simulink model "AXI_QPSK_Tx"  (R2020a)
settings: Solver=FixedStepAuto  StartTime=0.0  StopTime=1000/Rb  RelTol=1e-3
PreLoadFcn:
  | Rb = 1000;   % 1kbit / s
  | Rsym = Rb/2;   % 2 bits per symbol
  | Rsymbol = Rb/2;
  | OSR = 32;
  | f_error = 120;
  | 
  | design_filters_tx
undefined symbols (not defined in the file or in its folder): AXI4, CIC_fine_Tx, fCIC, fHB, Lite, R_CIC, R_CICcomp, R_HB, R_RRC
libraries: xbsIndex_r4 x281, hdlsllib x2
(part 1 of 3)
CloseFcn:
  | clear
settings Model: Creator=nas07122  LastModifiedBy=david
settings DataIOCC: ReturnWorkspaceOutputs=off
settings DebuggingCC: ArithmeticOperatorsInVariantConditions=warning
settings SFSimCC: SimUseLocalCustomCode=off  CustomCodeUndefinedFunction=UseInterfaceOnly
settings RTWCC: RTWUseLocalCustomCode=off
settings CodeAppCC: StateflowObjectComments=on

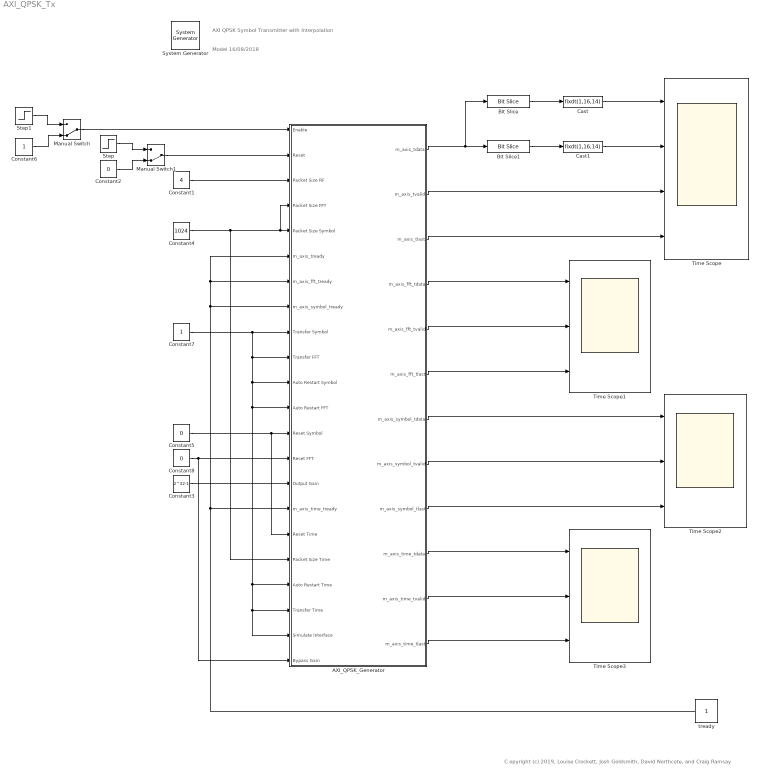
== system AXI_QPSK_Tx ==
  note: Model 16/08/2018
  note: AXI QPSK Symbol Transmitter with Interpolation
  note: C opyright (c) 2019, Louise Crockett, Josh Goldsmith, David Northcote, and Craig Ramsay
  " System Generator" : xbsIndex_r4/ System Generator  Tag=genX  xilinxfamily=zynquplusRFSOC  part=xczu28dr  speed=-2-e  package=ffvg1517  synthesis_tool=Vivado  clock_wrapper=Clock Enables  directory=../iprepo/zcu111/tx  proj_type=Vivado  Synth_file=Vivado Synthesis Defaults  Impl_file=Vivado Implementation Defaults  testbench=off  simulink_period=1/(0.5*Rb*R_RRC*R_HB*R_CICcomp*R_CIC)  sysclk_period=(1/fCIC)*1e9  dcm_input_clock_period=10  incr_netlist=off  trim_vbits=Everywhere in SubSystem  dbl_ovrd=According to Block Masks  core_generation=According to Block Masks  run_coregen=off  deprecated_control=off  eval_field=0  block_type=sysgen
  AXI_QPSK_Generator : Subsystem
  Bit Slice : hdlsllib/Logic and Bit Operations/Bit Slice  lidx=15  ridx=0
      settings: SourceProductBaseCode=SL
  Bit Slice1 : hdlsllib/Logic and Bit Operations/Bit Slice  lidx=31  ridx=16
      settings: SourceProductBaseCode=SL
  Cast : DataTypeConversion  OutDataTypeStr=fixdt(1,16,14)  ConvertRealWorld=Stored Integer (SI)
  Cast1 : DataTypeConversion  OutDataTypeStr=fixdt(1,16,14)  ConvertRealWorld=Stored Integer (SI)
  Constant1 : Constant  Value=4  SampleTime=2/Rb
  Constant2 : Constant  Value=0  SampleTime=2/Rb
  Constant3 : Constant  Value=2^32-1  SampleTime=1/fHB
  Constant4 : Constant  Value=1024  SampleTime=1/fCIC
  Constant5 : Constant  Value=0  SampleTime=1/fCIC
  Constant6 : Constant  SampleTime=2/Rb
  Constant7 : Constant  SampleTime=1/fCIC
  Constant8 : Constant  Value=0  SampleTime=1/fHB
  Manual Switch : ManualSwitch  CurrentSetting=0
  Manual Switch1 : ManualSwitch  CurrentSetting=0
  Step : Step  Time=5/Rb  Before=1  After=0  SampleTime=2/Rb
  Step1 : Step  Time=8/Rb  SampleTime=2/Rb
  Time Scope : Scope  NumInputPorts=4
  Time Scope1 : Scope  NumInputPorts=3
  Time Scope2 : Scope  NumInputPorts=3
  Time Scope3 : Scope  NumInputPorts=3
  tready : Constant  VectorParams1D=off  OutDataTypeStr=boolean  SampleTime=-1
  wires:
  Step1/1 -> Manual Switch/1
  Constant6/1 -> Manual Switch/2
  Bit Slice/1 -> Cast/1
  Bit Slice1/1 -> Cast1/1
  AXI_QPSK_Generator/1(m_axis_tdata) -> Bit Slice/1, Bit Slice1/1
  Manual Switch/1 -> AXI_QPSK_Generator/1(Enable)
  Constant1/1 -> AXI_QPSK_Generator/3(Packet Size RF)
  tready/1 -> AXI_QPSK_Generator/6(m_axis_tready), AXI_QPSK_Generator/7(m_axis_fft_tready), AXI_QPSK_Generator/8(m_axis_symbol_tready), AXI_QPSK_Generator/16(m_axis_time_tready)
  AXI_QPSK_Generator/2(m_axis_tvalid) -> Time Scope/3
  AXI_QPSK_Generator/3(m_axis_tlast) -> Time Scope/4
  Cast1/1 -> Time Scope/2
  Cast/1 -> Time Scope/1
  Manual Switch1/1 -> AXI_QPSK_Generator/2(Reset)
  Step/1 -> Manual Switch1/1
  Constant2/1 -> Manual Switch1/2
  Constant4/1 -> AXI_QPSK_Generator/4(Packet Size FFT), AXI_QPSK_Generator/5(Packet Size Symbol), AXI_QPSK_Generator/18(Packet Size Time)
  AXI_QPSK_Generator/7(m_axis_symbol_tdata) -> Time Scope2/1
  AXI_QPSK_Generator/8(m_axis_symbol_tvalid) -> Time Scope2/2
  AXI_QPSK_Generator/9(m_axis_symbol_tlast) -> Time Scope2/3
  AXI_QPSK_Generator/6(m_axis_fft_tlast) -> Time Scope1/3
  AXI_QPSK_Generator/5(m_axis_fft_tvalid) -> Time Scope1/2
  AXI_QPSK_Generator/4(m_axis_fft_tdata) -> Time Scope1/1
  Constant5/1 -> AXI_QPSK_Generator/17(Reset Time), AXI_QPSK_Generator/13(Reset Symbol)
  Constant7/1 -> AXI_QPSK_Generator/21(Simulate Interface), AXI_QPSK_Generator/20(Transfer Time), AXI_QPSK_Generator/19(Auto Restart Time), AXI_QPSK_Generator/12(Auto Restart FFT), AXI_QPSK_Generator/11(Auto Restart Symbol), AXI_QPSK_Generator/10(Transfer FFT), AXI_QPSK_Generator/9(Transfer Symbol)
  Constant8/1 -> AXI_QPSK_Generator/22(Bypass Gain), AXI_QPSK_Generator/14(Reset FFT)
  AXI_QPSK_Generator/10(m_axis_time_tdata) -> Time Scope3/1
  AXI_QPSK_Generator/11(m_axis_time_tvalid) -> Time Scope3/2
  AXI_QPSK_Generator/12(m_axis_time_tlast) -> Time Scope3/3
  Constant3/1 -> AXI_QPSK_Generator/15(Output Gain)

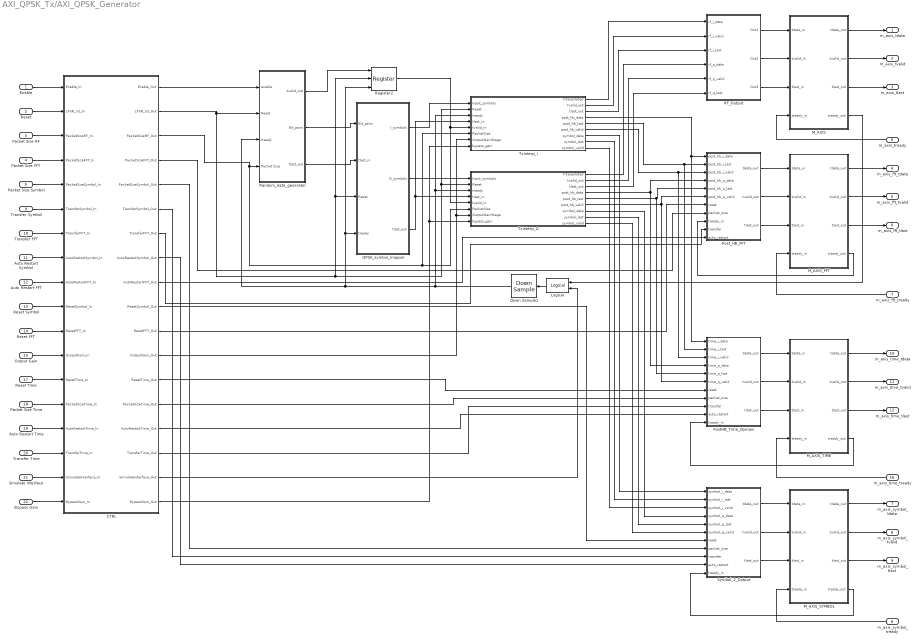
== system AXI_QPSK_Tx/AXI_QPSK_Generator ==
  Enable : Inport
  Reset : Inport  Port=2
  Packet Size RF : Inport  Port=3
  Packet Size FFT : Inport  Port=4
  Packet Size Symbol : Inport  Port=5
  m_axis_tready : Inport  Port=6
  m_axis_fft_tready : Inport  Port=7
  m_axis_symbol_tready : Inport  Port=8
  Transfer Symbol : Inport  Port=9
  Transfer FFT : Inport  Port=10
  Auto Restart Symbol : Inport  Port=11
  Auto Restart FFT : Inport  Port=12
  Reset Symbol : Inport  Port=13
  Reset FFT : Inport  Port=14
  Output Gain : Inport  Port=15
  m_axis_time_tready : Inport  Port=16
  Reset Time : Inport  Port=17
  Packet Size Time : Inport  Port=18
  Auto Restart Time : Inport  Port=19
  Transfer Time : Inport  Port=20
  Simulate Interface : Inport  Port=21
  Bypass Gain : Inport  Port=22
  CTRL : Subsystem
  Down Sample1 : xbsIndex_r4/Down Sample  sample_ratio=fCIC/(Rb/2)  sample_phase=First Value of Frame  en=off  rst=off  latency=0  dbl_ovrd=off  block_type=dsamp
  Logical : xbsIndex_r4/Logical  logical_function=OR  inputs=2  en=off  latency=0  precision=Full  arith_type=Unsigned  n_bits=16  bin_pt=0  align_bp=on  dbl_ovrd=off  block_type=logical
  M_AXIS : Subsystem
  M_AXIS_FFT : Subsystem
  M_AXIS_SYMBOL : Subsystem
  M_AXIS_TIME : Subsystem
  PostHB_Time_Domain : Subsystem
  Post_HB_FFT : Subsystem
  QPSK_symbol_mapper : Subsystem
  RF_Output : Subsystem
  Random_data_generator : Subsystem
  Register2 : xbsIndex_r4/Register  init=0  rst=on  en=on  dbl_ovrd=off  block_type=register
  Symbol_2_Output : Subsystem
  TxInterp_I : Subsystem
  TxInterp_Q : Subsystem
  m_axis_tdata : Outport  VectorParamsAs1DForOutWhenUnconnected=off
  m_axis_tvalid : Outport  Port=2  VectorParamsAs1DForOutWhenUnconnected=off
  m_axis_tlast : Outport  Port=3  VectorParamsAs1DForOutWhenUnconnected=off
  m_axis_fft_tdata : Outport  Port=4  VectorParamsAs1DForOutWhenUnconnected=off
  m_axis_fft_tvalid : Outport  Port=5  VectorParamsAs1DForOutWhenUnconnected=off
  m_axis_fft_tlast : Outport  Port=6  VectorParamsAs1DForOutWhenUnconnected=off
  m_axis_symbol_tdata : Outport  Port=7  VectorParamsAs1DForOutWhenUnconnected=off
  m_axis_symbol_tvalid : Outport  Port=8  VectorParamsAs1DForOutWhenUnconnected=off
  m_axis_symbol_tlast : Outport  Port=9  VectorParamsAs1DForOutWhenUnconnected=off
  m_axis_time_tdata : Outport  Port=10  VectorParamsAs1DForOutWhenUnconnected=off
  m_axis_time_tvalid : Outport  Port=11  VectorParamsAs1DForOutWhenUnconnected=off
  m_axis_time_tlast : Outport  Port=12  VectorParamsAs1DForOutWhenUnconnected=off
  wires:
  QPSK_symbol_mapper/3(tlast_out) -> TxInterp_I/4(tlast_in), TxInterp_Q/4(tlast_in)
  M_AXIS/2(tvalid_out) -> m_axis_tvalid/1
  QPSK_symbol_mapper/1(I_symbols) -> TxInterp_I/1(Input_symbols)
  m_axis_tready/1 -> M_AXIS/4(tready_in)
  QPSK_symbol_mapper/2(Q_symbols) -> TxInterp_Q/1(Input_symbols)
  Packet Size RF/1 -> CTRL/3(PacketSizeRF_In)
  Reset/1 -> CTRL/2(LFSR_rst_In)
  Random_data_generator/3(tlast_out) -> QPSK_symbol_mapper/2(tlast_in)
  Enable/1 -> CTRL/1(Enable_In)
  Random_data_generator/2(Bit_pairs) -> QPSK_symbol_mapper/1(Bit_pairs)
  CTRL/3(PacketSizeRF_Out) -> TxInterp_I/6(PacketSize), TxInterp_Q/6(PacketSize), Random_data_generator/4(Packet Size)
  M_AXIS/3(tlast_out) -> m_axis_tlast/1
  M_AXIS/1(tdata_out) -> m_axis_tdata/1
  Down Sample1/1 -> Random_data_generator/3(tready), Register2/3, QPSK_symbol_mapper/4(tready), TxInterp_I/3(tready), TxInterp_Q/3(tready)
  CTRL/2(LFSR_rst_Out) -> TxInterp_I/2(Reset), TxInterp_Q/2(Reset), QPSK_symbol_mapper/3(Reset), Register2/2, Random_data_generator/2(Reset)
  CTRL/1(Enable_Out) -> Random_data_generator/1(enable)
  Random_data_generator/1(tvalid_out) -> Register2/1
  Register2/1 -> TxInterp_I/5(tvalid_in), TxInterp_Q/5(tvalid_in)
  Post_HB_FFT/1(tdata_out) -> M_AXIS_FFT/1(tdata_in)
  Post_HB_FFT/2(tvalid_out) -> M_AXIS_FFT/2(tvalid_in)
  Post_HB_FFT/3(tlast_out) -> M_AXIS_FFT/3(tlast_in)
  M_AXIS_FFT/1(tdata_out) -> m_axis_fft_tdata/1
  M_AXIS_FFT/3(tlast_out) -> m_axis_fft_tlast/1
  m_axis_fft_tready/1 -> M_AXIS_FFT/4(tready_in)
  M_AXIS_FFT/2(tvalid_out) -> m_axis_fft_tvalid/1
  M_AXIS_SYMBOL/2(tvalid_out) -> m_axis_symbol_tvalid/1
  m_axis_symbol_tready/1 -> M_AXIS_SYMBOL/4(tready_in)
  M_AXIS_SYMBOL/3(tlast_out) -> m_axis_symbol_tlast/1
  M_AXIS_SYMBOL/1(tdata_out) -> m_axis_symbol_tdata/1
  TxInterp_I/4(post_hb_data) -> PostHB_Time_Domain/1(time_i_data), Post_HB_FFT/1(post_hb_i_data)
  TxInterp_I/5(post_hb_last) -> PostHB_Time_Domain/2(time_i_last), Post_HB_FFT/2(post_hb_i_last)
  TxInterp_I/6(post_hb_valid) -> PostHB_Time_Domain/3(time_i_valid), Post_HB_FFT/3(post_hb_i_valid)
  Symbol_2_Output/1(tdata_out) -> M_AXIS_SYMBOL/1(tdata_in)
  Symbol_2_Output/2(tvalid_out) -> M_AXIS_SYMBOL/2(tvalid_in)
  Symbol_2_Output/3(tlast_out) -> M_AXIS_SYMBOL/3(tlast_in)
  M_AXIS_SYMBOL/4(tready_out) -> Symbol_2_Output/11(tready_in)
  M_AXIS_FFT/4(tready_out) -> Post_HB_FFT/9(tready_in)
  TxInterp_I/1(Interpolated) -> RF_Output/1(rf_i_data)
  TxInterp_I/2(tvalid_out) -> RF_Output/2(rf_i_valid)
  TxInterp_I/3(tlast_out) -> RF_Output/3(rf_i_last)
  RF_Output/1(Out1) -> M_AXIS/1(tdata_in)
  RF_Output/2(Out2) -> M_AXIS/2(tvalid_in)
  RF_Output/3(Out3) -> M_AXIS/3(tlast_in)
  TxInterp_I/7(symbol_data) -> Symbol_2_Output/1(symbol_i_data)
  TxInterp_I/8(symbol_last) -> Symbol_2_Output/2(symbol_i_last)
  TxInterp_I/9(symbol_valid) -> Symbol_2_Output/3(symbol_i_valid)
  CTRL/4(PacketSizeFFT_Out) -> Post_HB_FFT/8(packet_size)
  CTRL/5(PacketSizeSymbol_Out) -> Symbol_2_Output/8(packet_size)
  Packet Size FFT/1 -> CTRL/4(PacketSizeFFT_In)
  Packet Size Symbol/1 -> CTRL/5(PacketSizeSymbol_In)
  CTRL/6(TransferSymbol_Out) -> Symbol_2_Output/9(transfer)
  CTRL/8(AutoRestartSymbol_Out) -> Symbol_2_Output/10(auto_restart)
  CTRL/10(ResetSymbol_Out) -> Symbol_2_Output/7(reset)
  Transfer Symbol/1 -> CTRL/6(TransferSymbol_In)
  Transfer FFT/1 -> CTRL/7(TransferFFT_In)
  Auto Restart Symbol/1 -> CTRL/8(AutoRestartSymbol_In)
  Auto Restart FFT/1 -> CTRL/9(AutoRestartFFT_In)
  Reset Symbol/1 -> CTRL/10(ResetSymbol_In)
  Reset FFT/1 -> CTRL/11(ResetFFT_In)
  CTRL/7(TransferFFT_Out) -> Post_HB_FFT/10(transfer)
  CTRL/9(AutoRestartFFT_Out) -> Post_HB_FFT/11(auto_restart)
  CTRL/11(ResetFFT_Out) -> Post_HB_FFT/7(reset)
  CTRL/12(OutputGain_Out) -> TxInterp_I/7(OutputGainStage), TxInterp_Q/7(OutputGainStage)
  Output Gain/1 -> CTRL/12(OutputGain_In)
  M_AXIS_TIME/4(tready_out) -> PostHB_Time_Domain/11(tready_in)
  PostHB_Time_Domain/3(tlast_out) -> M_AXIS_TIME/3(tlast_in)
  PostHB_Time_Domain/2(tvalid_out) -> M_AXIS_TIME/2(tvalid_in)
  PostHB_Time_Domain/1(tdata_out) -> M_AXIS_TIME/1(tdata_in)
  M_AXIS_TIME/1(tdata_out) -> m_axis_time_tdata/1
  M_AXIS_TIME/3(tlast_out) -> m_axis_time_tlast/1
  m_axis_time_tready/1 -> M_AXIS_TIME/4(tready_in)
  M_AXIS_TIME/2(tvalid_out) -> m_axis_time_tvalid/1
  CTRL/13(ResetTime_Out) -> PostHB_Time_Domain/7(reset)
  CTRL/14(PacketSizeTime_Out) -> PostHB_Time_Domain/8(packet_size)
  CTRL/15(AutoRestartTime_Out) -> PostHB_Time_Domain/10(auto_restart)
  CTRL/16(TransferTime_Out) -> PostHB_Time_Domain/9(transfer)
  Reset Time/1 -> CTRL/13(ResetTime_In)
  Packet Size Time/1 -> CTRL/14(PacketSizeTime_In)
  Auto Restart Time/1 -> CTRL/15(AutoRestartTime_In)
  Transfer Time/1 -> CTRL/16(TransferTime_In)
  M_AXIS/4(tready_out) -> Logical/1
  Logical/1 -> Down Sample1/1
  CTRL/17(SimulateInterface_Out) -> Logical/2
  Simulate Interface/1 -> CTRL/17(SimulateInterface_In)
  CTRL/18(BypassGain_Out) -> TxInterp_I/8(bypass_gain), TxInterp_Q/8(bypass_gain)
  TxInterp_Q/1(Interpolated) -> RF_Output/4(rf_q_data)
  TxInterp_Q/2(tvalid_out) -> RF_Output/5(rf_q_valid)
  TxInterp_Q/3(tlast_out) -> RF_Output/6(rf_q_last)
  TxInterp_Q/4(post_hb_data) -> PostHB_Time_Domain/4(time_q_data), Post_HB_FFT/4(post_hb_q_data)
  TxInterp_Q/5(post_hb_last) -> PostHB_Time_Domain/5(time_q_last), Post_HB_FFT/5(post_hb_q_last)
  TxInterp_Q/6(post_hb_valid) -> PostHB_Time_Domain/6(time_q_valid), Post_HB_FFT/6(post_hb_q_valid)
  TxInterp_Q/7(symbol_data) -> Symbol_2_Output/4(symbol_q_data)
  TxInterp_Q/8(symbol_last) -> Symbol_2_Output/5(symbol_q_last)
  TxInterp_Q/9(symbol_valid) -> Symbol_2_Output/6(symbol_q_valid)
  Bypass Gain/1 -> CTRL/18(BypassGain_In)

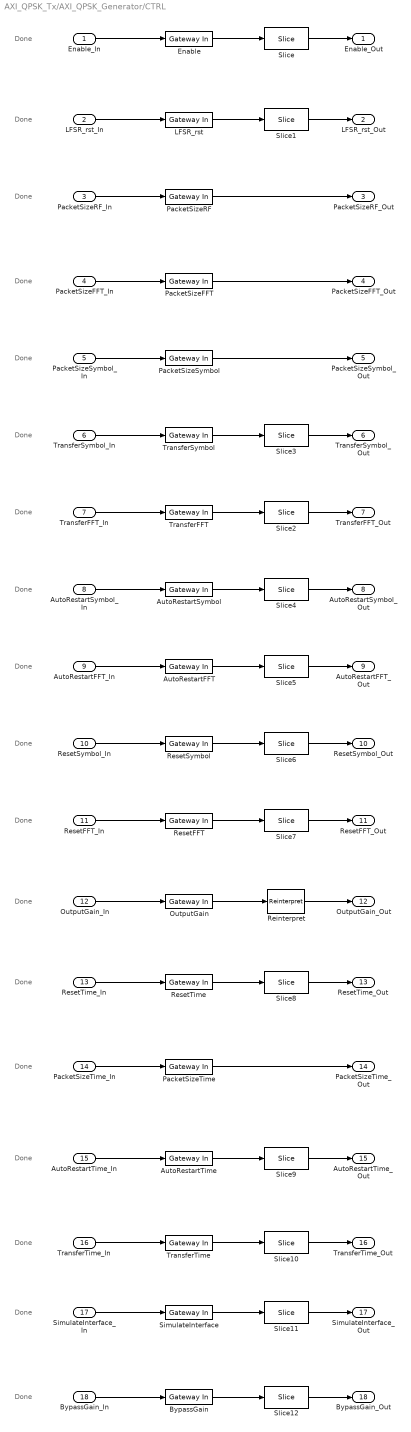
== system AXI_QPSK_Tx/AXI_QPSK_Generator/CTRL ==
  note: Done
  note: Done
  note: Done
  note: Done
  note: Done
  note: Done
  note: Done
  note: Done
  note: Done
  note: Done
  note: Done
  note: Done
  note: Done
  note: Done
  note: Done
  note: Done
  note: Done
  note: Done
  Enable_In : Inport
  LFSR_rst_In : Inport  Port=2
  PacketSizeRF_In : Inport  Port=3
  PacketSizeFFT_In : Inport  Port=4
  PacketSizeSymbol_In : Inport  Port=5
  TransferSymbol_In : Inport  Port=6
  TransferFFT_In : Inport  Port=7
  AutoRestartSymbol_In : Inport  Port=8
  AutoRestartFFT_In : Inport  Port=9
  ResetSymbol_In : Inport  Port=10
  ResetFFT_In : Inport  Port=11
  OutputGain_In : Inport  Port=12
  ResetTime_In : Inport  Port=13
  PacketSizeTime_In : Inport  Port=14
  AutoRestartTime_In : Inport  Port=15
  TransferTime_In : Inport  Port=16
  SimulateInterface_In : Inport  Port=17
  BypassGain_In : Inport  Port=18
  AutoRestartFFT : xbsIndex_r4/Gateway In  gui_display_data_type=Fixed-point  arith_type=Unsigned  n_bits=32  bin_pt=0  preci_type=Single  exp_width=8  frac_width=24  rows=1  columns=1  quantization=Truncate  overflow=Wrap  period=1/fCIC  UseAsADC=off  ADCChannel='1'  interface=AXI4-Lite  automatic_assignment=off  address_offset=40  intf_name=''  intf_description=''  default_value=0  timing_constraint=None  locs_specified=off  LOCs={}  io_standard={}  inherit_from_input=off  hdl_port=on  dbl_ovrd=off  block_type=gatewayin
  AutoRestartSymbol : xbsIndex_r4/Gateway In  gui_display_data_type=Fixed-point  arith_type=Unsigned  n_bits=32  bin_pt=0  preci_type=Single  exp_width=8  frac_width=24  rows=1  columns=1  quantization=Truncate  overflow=Wrap  period=1/fCIC  UseAsADC=off  ADCChannel='1'  interface=AXI4-Lite  automatic_assignment=off  address_offset=36  intf_name=''  intf_description=''  default_value=0  timing_constraint=None  locs_specified=off  LOCs={}  io_standard={}  inherit_from_input=off  hdl_port=on  dbl_ovrd=off  block_type=gatewayin
  AutoRestartTime : xbsIndex_r4/Gateway In  gui_display_data_type=Fixed-point  arith_type=Unsigned  n_bits=32  bin_pt=0  preci_type=Single  exp_width=8  frac_width=24  rows=1  columns=1  quantization=Truncate  overflow=Wrap  period=1/fCIC  UseAsADC=off  ADCChannel='1'  interface=AXI4-Lite  automatic_assignment=off  address_offset=56  intf_name=''  intf_description=''  default_value=0  timing_constraint=None  locs_specified=off  LOCs={}  io_standard={}  inherit_from_input=off  hdl_port=on  dbl_ovrd=off  block_type=gatewayin
  BypassGain : xbsIndex_r4/Gateway In  gui_display_data_type=Fixed-point  arith_type=Unsigned  n_bits=32  bin_pt=0  preci_type=Single  exp_width=8  frac_width=24  rows=1  columns=1  quantization=Truncate  overflow=Wrap  period=1/fHB  UseAsADC=off  ADCChannel='1'  interface=AXI4-Lite  automatic_assignment=off  address_offset=68  intf_name=''  intf_description=''  default_value=0  timing_constraint=None  locs_specified=off  LOCs={}  io_standard={}  inherit_from_input=off  hdl_port=on  dbl_ovrd=off  block_type=gatewayin
  Enable : xbsIndex_r4/Gateway In  gui_display_data_type=Fixed-point  arith_type=Unsigned  n_bits=32  bin_pt=0  preci_type=Single  exp_width=8  frac_width=24  rows=1  columns=1  quantization="Round  (unbiased: +/- Inf)"  overflow=Saturate  period=2/Rb  UseAsADC=off  ADCChannel='1'  interface=AXI4-Lite  automatic_assignment=off  address_offset=32  intf_name=''  intf_description=''  default_value=0  timing_constraint=None  locs_specified=off  LOCs={}  io_standard={}  inherit_from_input=off  hdl_port=on  dbl_ovrd=off  block_type=gatewayin
  LFSR_rst : xbsIndex_r4/Gateway In  gui_display_data_type=Fixed-point  arith_type=Unsigned  n_bits=32  bin_pt=0  preci_type=Single  exp_width=8  frac_width=24  rows=1  columns=1  quantization="Round  (unbiased: +/- Inf)"  overflow=Saturate  period=2/Rb  UseAsADC=off  ADCChannel='1'  interface=AXI4-Lite  automatic_assignment=off  address_offset=28  intf_name=''  intf_description=''  default_value=0  timing_constraint=None  locs_specified=off  LOCs={}  io_standard={}  inherit_from_input=off  hdl_port=on  dbl_ovrd=off  block_type=gatewayin
  OutputGain : xbsIndex_r4/Gateway In  gui_display_data_type=Fixed-point  arith_type=Unsigned  n_bits=32  bin_pt=0  preci_type=Single  exp_width=8  frac_width=24  rows=1  columns=1  quantization=Truncate  overflow=Wrap  period=1/fHB  UseAsADC=off  ADCChannel='1'  interface=AXI4-Lite  automatic_assignment=off  address_offset=44  intf_name=''  intf_description=''  default_value=0  timing_constraint=None  locs_specified=off  LOCs={}  io_standard={}  inherit_from_input=off  hdl_port=on  dbl_ovrd=off  block_type=gatewayin
  PacketSizeFFT : xbsIndex_r4/Gateway In  gui_display_data_type=Fixed-point  arith_type=Unsigned  n_bits=32  bin_pt=0  preci_type=Single  exp_width=8  frac_width=24  rows=1  columns=1  quantization=Truncate  overflow=Wrap  period=1/fCIC  UseAsADC=off  ADCChannel='1'  interface=AXI4-Lite  automatic_assignment=off  address_offset=24  intf_name=''  intf_description=''  default_value=0  timing_constraint=None  locs_specified=off  LOCs={}  io_standard={}  inherit_from_input=off  hdl_port=on  dbl_ovrd=off  block_type=gatewayin
  PacketSizeRF : xbsIndex_r4/Gateway In  gui_display_data_type=Fixed-point  arith_type=Unsigned  n_bits=32  bin_pt=0  preci_type=Single  exp_width=8  frac_width=24  rows=1  columns=1  quantization=Truncate  overflow=Wrap  period=2/Rb  UseAsADC=off  ADCChannel='1'  interface=AXI4-Lite  automatic_assignment=off  address_offset=20  intf_name=''  intf_description=''  default_value=0  timing_constraint=None  locs_specified=off  LOCs={}  io_standard={}  inherit_from_input=off  hdl_port=on  dbl_ovrd=off  block_type=gatewayin
  PacketSizeSymbol : xbsIndex_r4/Gateway In  gui_display_data_type=Fixed-point  arith_type=Unsigned  n_bits=32  bin_pt=0  preci_type=Single  exp_width=8  frac_width=24  rows=1  columns=1  quantization=Truncate  overflow=Wrap  period=1/fCIC  UseAsADC=off  ADCChannel='1'  interface=AXI4-Lite  automatic_assignment=off  address_offset=16  intf_name=''  intf_description=''  default_value=0  timing_constraint=None  locs_specified=off  LOCs={}  io_standard={}  inherit_from_input=off  hdl_port=on  dbl_ovrd=off  block_type=gatewayin
  PacketSizeTime : xbsIndex_r4/Gateway In  gui_display_data_type=Fixed-point  arith_type=Unsigned  n_bits=32  bin_pt=0  preci_type=Single  exp_width=8  frac_width=24  rows=1  columns=1  quantization=Truncate  overflow=Wrap  period=1/fCIC  UseAsADC=off  ADCChannel='1'  interface=AXI4-Lite  automatic_assignment=off  address_offset=52  intf_name=''  intf_description=''  default_value=0  timing_constraint=None  locs_specified=off  LOCs={}  io_standard={}  inherit_from_input=off  hdl_port=on  dbl_ovrd=off  block_type=gatewayin
  Reinterpret : xbsIndex_r4/Reinterpret  force_arith_type=off  arith_type=Unsigned  force_bin_pt=on  bin_pt=32  block_type=reinterpret
  ResetFFT : xbsIndex_r4/Gateway In  gui_display_data_type=Fixed-point  arith_type=Unsigned  n_bits=32  bin_pt=0  preci_type=Single  exp_width=8  frac_width=24  rows=1  columns=1  quantization=Truncate  overflow=Wrap  period=1/fHB  UseAsADC=off  ADCChannel='1'  interface=AXI4-Lite  automatic_assignment=off  address_offset=12  intf_name=''  intf_description=''  default_value=0  timing_constraint=None  locs_specified=off  LOCs={}  io_standard={}  inherit_from_input=off  hdl_port=on  dbl_ovrd=off  block_type=gatewayin
  ResetSymbol : xbsIndex_r4/Gateway In  gui_display_data_type=Fixed-point  arith_type=Unsigned  n_bits=32  bin_pt=0  preci_type=Single  exp_width=8  frac_width=24  rows=1  columns=1  quantization=Truncate  overflow=Wrap  period=1/fCIC  UseAsADC=off  ADCChannel='1'  interface=AXI4-Lite  automatic_assignment=off  address_offset=8  intf_name=''  intf_description=''  default_value=0  timing_constraint=None  locs_specified=off  LOCs={}  io_standard={}  inherit_from_input=off  hdl_port=on  dbl_ovrd=off  block_type=gatewayin
  ResetTime : xbsIndex_r4/Gateway In  gui_display_data_type=Fixed-point  arith_type=Unsigned  n_bits=32  bin_pt=0  preci_type=Single  exp_width=8  frac_width=24  rows=1  columns=1  quantization=Truncate  overflow=Wrap  period=1/fCIC  UseAsADC=off  ADCChannel='1'  interface=AXI4-Lite  automatic_assignment=off  address_offset=48  intf_name=''  intf_description=''  default_value=0  timing_constraint=None  locs_specified=off  LOCs={}  io_standard={}  inherit_from_input=off  hdl_port=on  dbl_ovrd=off  block_type=gatewayin
  SimulateInterface : xbsIndex_r4/Gateway In  gui_display_data_type=Fixed-point  arith_type=Unsigned  n_bits=32  bin_pt=0  preci_type=Single  exp_width=8  frac_width=24  rows=1  columns=1  quantization=Truncate  overflow=Wrap  period=1/fCIC  UseAsADC=off  ADCChannel='1'  interface=AXI4-Lite  automatic_assignment=off  address_offset=64  intf_name=''  intf_description=''  default_value=0  timing_constraint=None  locs_specified=off  LOCs={}  io_standard={}  inherit_from_input=off  hdl_port=on  dbl_ovrd=off  block_type=gatewayin
  Slice{,1..12} (13 alike) : xbsIndex_r4/Slice  nbits=1  boolean_output=on  mode=Two Bit Locations  bit1=0  base1=LSB of Input  bit0=0  base0=LSB of Input  dbl_ovrd=off  block_type=slice
  TransferFFT : xbsIndex_r4/Gateway In  gui_display_data_type=Fixed-point  arith_type=Unsigned  n_bits=32  bin_pt=0  preci_type=Single  exp_width=8  frac_width=24  rows=1  columns=1  quantization=Truncate  overflow=Wrap  period=1/fCIC  UseAsADC=off  ADCChannel='1'  interface=AXI4-Lite  automatic_assignment=off  address_offset=4  intf_name=''  intf_description=''  default_value=0  timing_constraint=None  locs_specified=off  LOCs={}  io_standard={}  inherit_from_input=off  hdl_port=on  dbl_ovrd=off  block_type=gatewayin
  TransferSymbol : xbsIndex_r4/Gateway In  gui_display_data_type=Fixed-point  arith_type=Unsigned  n_bits=32  bin_pt=0  preci_type=Single  exp_width=8  frac_width=24  rows=1  columns=1  quantization=Truncate  overflow=Wrap  period=1/fCIC  UseAsADC=off  ADCChannel='1'  interface=AXI4-Lite  automatic_assignment=off  address_offset=0  intf_name=''  intf_description=''  default_value=0  timing_constraint=None  locs_specified=off  LOCs={}  io_standard={}  inherit_from_input=off  hdl_port=on  dbl_ovrd=off  block_type=gatewayin
  TransferTime : xbsIndex_r4/Gateway In  gui_display_data_type=Fixed-point  arith_type=Unsigned  n_bits=32  bin_pt=0  preci_type=Single  exp_width=8  frac_width=24  rows=1  columns=1  quantization=Truncate  overflow=Wrap  period=1/fCIC  UseAsADC=off  ADCChannel='1'  interface=AXI4-Lite  automatic_assignment=off  address_offset=60  intf_name=''  intf_description=''  default_value=0  timing_constraint=None  locs_specified=off  LOCs={}  io_standard={}  inherit_from_input=off  hdl_port=on  dbl_ovrd=off  block_type=gatewayin
  Enable_Out : Outport  VectorParamsAs1DForOutWhenUnconnected=off
  LFSR_rst_Out : Outport  Port=2  VectorParamsAs1DForOutWhenUnconnected=off
  PacketSizeRF_Out : Outport  Port=3  VectorParamsAs1DForOutWhenUnconnected=off
  PacketSizeFFT_Out : Outport  Port=4  VectorParamsAs1DForOutWhenUnconnected=off
  PacketSizeSymbol_Out : Outport  Port=5  VectorParamsAs1DForOutWhenUnconnected=off
  TransferSymbol_Out : Outport  Port=6  VectorParamsAs1DForOutWhenUnconnected=off
  TransferFFT_Out : Outport  Port=7  VectorParamsAs1DForOutWhenUnconnected=off
  AutoRestartSymbol_Out : Outport  Port=8  VectorParamsAs1DForOutWhenUnconnected=off
  AutoRestartFFT_Out : Outport  Port=9  VectorParamsAs1DForOutWhenUnconnected=off
  ResetSymbol_Out : Outport  Port=10  VectorParamsAs1DForOutWhenUnconnected=off
  ResetFFT_Out : Outport  Port=11  VectorParamsAs1DForOutWhenUnconnected=off
  OutputGain_Out : Outport  Port=12  VectorParamsAs1DForOutWhenUnconnected=off
  ResetTime_Out : Outport  Port=13  VectorParamsAs1DForOutWhenUnconnected=off
  PacketSizeTime_Out : Outport  Port=14  VectorParamsAs1DForOutWhenUnconnected=off
  AutoRestartTime_Out : Outport  Port=15  VectorParamsAs1DForOutWhenUnconnected=off
  TransferTime_Out : Outport  Port=16  VectorParamsAs1DForOutWhenUnconnected=off
  SimulateInterface_Out : Outport  Port=17  VectorParamsAs1DForOutWhenUnconnected=off
  BypassGain_Out : Outport  Port=18  VectorParamsAs1DForOutWhenUnconnected=off
  wires:
  Enable/1 -> Slice/1
  LFSR_rst_In/1 -> LFSR_rst/1
  LFSR_rst/1 -> Slice1/1
  PacketSizeRF_In/1 -> PacketSizeRF/1
  Enable_In/1 -> Enable/1
  Slice/1 -> Enable_Out/1
  Slice1/1 -> LFSR_rst_Out/1
  PacketSizeRF/1 -> PacketSizeRF_Out/1
  PacketSizeFFT/1 -> PacketSizeFFT_Out/1
  PacketSizeFFT_In/1 -> PacketSizeFFT/1
  PacketSizeSymbol_In/1 -> PacketSizeSymbol/1
  PacketSizeSymbol/1 -> PacketSizeSymbol_Out/1
  TransferFFT/1 -> Slice2/1
  TransferFFT_In/1 -> TransferFFT/1
  TransferSymbol_In/1 -> TransferSymbol/1
  TransferSymbol/1 -> Slice3/1
  AutoRestartSymbol/1 -> Slice4/1
  AutoRestartSymbol_In/1 -> AutoRestartSymbol/1
  AutoRestartFFT_In/1 -> AutoRestartFFT/1
  AutoRestartFFT/1 -> Slice5/1
  Slice2/1 -> TransferFFT_Out/1
  Slice3/1 -> TransferSymbol_Out/1
  Slice4/1 -> AutoRestartSymbol_Out/1
  Slice5/1 -> AutoRestartFFT_Out/1
  ResetFFT/1 -> Slice7/1
  ResetFFT_In/1 -> ResetFFT/1
  ResetSymbol_In/1 -> ResetSymbol/1
  ResetSymbol/1 -> Slice6/1
  Slice6/1 -> ResetSymbol_Out/1
  Slice7/1 -> ResetFFT_Out/1
  OutputGain/1 -> Reinterpret/1
  OutputGain_In/1 -> OutputGain/1
  Slice8/1 -> ResetTime_Out/1
  ResetTime_In/1 -> ResetTime/1
  ResetTime/1 -> Slice8/1
  Slice9/1 -> AutoRestartTime_Out/1
  AutoRestartTime_In/1 -> AutoRestartTime/1
  AutoRestartTime/1 -> Slice9/1
  Slice10/1 -> TransferTime_Out/1
  TransferTime/1 -> Slice10/1
  TransferTime_In/1 -> TransferTime/1
  PacketSizeTime/1 -> PacketSizeTime_Out/1
  PacketSizeTime_In/1 -> PacketSizeTime/1
  Reinterpret/1 -> OutputGain_Out/1
  SimulateInterface_In/1 -> SimulateInterface/1
  SimulateInterface/1 -> Slice11/1
  Slice11/1 -> SimulateInterface_Out/1
  Slice12/1 -> BypassGain_Out/1
  BypassGain/1 -> Slice12/1
  BypassGain_In/1 -> BypassGain/1

== system AXI_QPSK_Tx/AXI_QPSK_Generator/M_AXIS ==
  tdata_in : Inport
  tvalid_in : Inport  Port=2
  tlast_in : Inport  Port=3
  tready_in : Inport  Port=4
  m_rf_axis_tdata : xbsIndex_r4/Gateway Out  inherit_from_input=on  hdl_port=on  rows=1  columns=1  UseAsDAC=off  DACChannel='1'  interface=None  automatic_assignment=on  address_offset=hex2dec('00')  intf_name=''  intf_description=''  timing_constraint=None  locs_specified=off  LOCs={}  io_standard={}  block_type=gatewayout
  m_rf_axis_tlast : xbsIndex_r4/Gateway Out  inherit_from_input=off  hdl_port=on  rows=1  columns=1  UseAsDAC=off  DACChannel='1'  interface=None  automatic_assignment=on  address_offset=hex2dec('00')  intf_name=''  intf_description=''  timing_constraint=None  locs_specified=off  LOCs={}  io_standard={}  block_type=gatewayout
  m_rf_axis_tready : xbsIndex_r4/Gateway In  gui_display_data_type=Boolean  arith_type=Boolean  n_bits=16  bin_pt=14  preci_type=Single  exp_width=8  frac_width=24  rows=1  columns=1  quantization="Round  (unbiased: +/- Inf)"  overflow=Saturate  period=1/(fCIC)  UseAsADC=off  ADCChannel='1'  interface=None  automatic_assignment=on  address_offset=hex2dec('00')  intf_name=''  intf_description=''  default_value=0  timing_constraint=None  locs_specified=off  LOCs={}  io_standard={}  inherit_from_input=off  hdl_port=on  dbl_ovrd=off  block_type=gatewayin
  m_rf_axis_tvalid : xbsIndex_r4/Gateway Out  inherit_from_input=off  hdl_port=on  rows=1  columns=1  UseAsDAC=off  DACChannel='1'  interface=None  automatic_assignment=on  address_offset=hex2dec('00')  intf_name=''  intf_description=''  timing_constraint=None  locs_specified=off  LOCs={}  io_standard={}  block_type=gatewayout
  tdata_out : Outport  VectorParamsAs1DForOutWhenUnconnected=off
  tvalid_out : Outport  Port=2  VectorParamsAs1DForOutWhenUnconnected=off
  tlast_out : Outport  Port=3  VectorParamsAs1DForOutWhenUnconnected=off
  tready_out : Outport  Port=4  VectorParamsAs1DForOutWhenUnconnected=off
  wires:
  tlast_in/1 -> m_rf_axis_tlast/1
  m_rf_axis_tlast/1 -> tlast_out/1
  m_rf_axis_tready/1 -> tready_out/1
  tvalid_in/1 -> m_rf_axis_tvalid/1
  m_rf_axis_tvalid/1 -> tvalid_out/1
  tdata_in/1 -> m_rf_axis_tdata/1
  m_rf_axis_tdata/1 -> tdata_out/1
  tready_in/1 -> m_rf_axis_tready/1

== system AXI_QPSK_Tx/AXI_QPSK_Generator/M_AXIS_FFT ==
  tdata_in : Inport
  tvalid_in : Inport  Port=2
  tlast_in : Inport  Port=3
  tready_in : Inport  Port=4
  m_fft_axis_tdata : xbsIndex_r4/Gateway Out  inherit_from_input=on  hdl_port=on  rows=1  columns=1  UseAsDAC=off  DACChannel='1'  interface=None  automatic_assignment=on  address_offset=hex2dec('00')  intf_name=''  intf_description=''  timing_constraint=None  locs_specified=off  LOCs={}  io_standard={}  block_type=gatewayout
  m_fft_axis_tlast : xbsIndex_r4/Gateway Out  inherit_from_input=off  hdl_port=on  rows=1  columns=1  UseAsDAC=off  DACChannel='1'  interface=None  automatic_assignment=on  address_offset=hex2dec('00')  intf_name=''  intf_description=''  timing_constraint=None  locs_specified=off  LOCs={}  io_standard={}  block_type=gatewayout
  m_fft_axis_tready : xbsIndex_r4/Gateway In  gui_display_data_type=Boolean  arith_type=Boolean  n_bits=16  bin_pt=14  preci_type=Single  exp_width=8  frac_width=24  rows=1  columns=1  quantization="Round  (unbiased: +/- Inf)"  overflow=Saturate  period=1/(fCIC)  UseAsADC=off  ADCChannel='1'  interface=None  automatic_assignment=on  address_offset=hex2dec('00')  intf_name=''  intf_description=''  default_value=0  timing_constraint=None  locs_specified=off  LOCs={}  io_standard={}  inherit_from_input=off  hdl_port=on  dbl_ovrd=off  block_type=gatewayin
  m_fft_axis_tvalid : xbsIndex_r4/Gateway Out  inherit_from_input=off  hdl_port=on  rows=1  columns=1  UseAsDAC=off  DACChannel='1'  interface=None  automatic_assignment=on  address_offset=hex2dec('00')  intf_name=''  intf_description=''  timing_constraint=None  locs_specified=off  LOCs={}  io_standard={}  block_type=gatewayout
  tdata_out : Outport  VectorParamsAs1DForOutWhenUnconnected=off
  tvalid_out : Outport  Port=2  VectorParamsAs1DForOutWhenUnconnected=off
  tlast_out : Outport  Port=3  VectorParamsAs1DForOutWhenUnconnected=off
  tready_out : Outport  Port=4  VectorParamsAs1DForOutWhenUnconnected=off
  wires:
  tready_in/1 -> m_fft_axis_tready/1
  m_fft_axis_tdata/1 -> tdata_out/1
  tdata_in/1 -> m_fft_axis_tdata/1
  m_fft_axis_tvalid/1 -> tvalid_out/1
  tvalid_in/1 -> m_fft_axis_tvalid/1
  m_fft_axis_tready/1 -> tready_out/1
  m_fft_axis_tlast/1 -> tlast_out/1
  tlast_in/1 -> m_fft_axis_tlast/1

== system AXI_QPSK_Tx/AXI_QPSK_Generator/M_AXIS_SYMBOL ==
  tdata_in : Inport
  tvalid_in : Inport  Port=2
  tlast_in : Inport  Port=3
  tready_in : Inport  Port=4
  m_symbol_axis_tdata : xbsIndex_r4/Gateway Out  inherit_from_input=on  hdl_port=on  rows=1  columns=1  UseAsDAC=off  DACChannel='1'  interface=None  automatic_assignment=on  address_offset=hex2dec('00')  intf_name=''  intf_description=''  timing_constraint=None  locs_specified=off  LOCs={}  io_standard={}  block_type=gatewayout
  m_symbol_axis_tlast : xbsIndex_r4/Gateway Out  inherit_from_input=off  hdl_port=on  rows=1  columns=1  UseAsDAC=off  DACChannel='1'  interface=None  automatic_assignment=on  address_offset=hex2dec('00')  intf_name=''  intf_description=''  timing_constraint=None  locs_specified=off  LOCs={}  io_standard={}  block_type=gatewayout
  m_symbol_axis_tready : xbsIndex_r4/Gateway In  gui_display_data_type=Boolean  arith_type=Boolean  n_bits=16  bin_pt=14  preci_type=Single  exp_width=8  frac_width=24  rows=1  columns=1  quantization="Round  (unbiased: +/- Inf)"  overflow=Saturate  period=1/(fCIC)  UseAsADC=off  ADCChannel='1'  interface=None  automatic_assignment=on  address_offset=hex2dec('00')  intf_name=''  intf_description=''  default_value=0  timing_constraint=None  locs_specified=off  LOCs={}  io_standard={}  inherit_from_input=off  hdl_port=on  dbl_ovrd=off  block_type=gatewayin
  m_symbol_axis_tvalid : xbsIndex_r4/Gateway Out  inherit_from_input=off  hdl_port=on  rows=1  columns=1  UseAsDAC=off  DACChannel='1'  interface=None  automatic_assignment=on  address_offset=hex2dec('00')  intf_name=''  intf_description=''  timing_constraint=None  locs_specified=off  LOCs={}  io_standard={}  block_type=gatewayout
  tdata_out : Outport  VectorParamsAs1DForOutWhenUnconnected=off
  tvalid_out : Outport  Port=2  VectorParamsAs1DForOutWhenUnconnected=off
  tlast_out : Outport  Port=3  VectorParamsAs1DForOutWhenUnconnected=off
  tready_out : Outport  Port=4  VectorParamsAs1DForOutWhenUnconnected=off
  wires:
  tlast_in/1 -> m_symbol_axis_tlast/1
  m_symbol_axis_tlast/1 -> tlast_out/1
  m_symbol_axis_tready/1 -> tready_out/1
  tvalid_in/1 -> m_symbol_axis_tvalid/1
  m_symbol_axis_tvalid/1 -> tvalid_out/1
  tdata_in/1 -> m_symbol_axis_tdata/1
  m_symbol_axis_tdata/1 -> tdata_out/1
  tready_in/1 -> m_symbol_axis_tready/1

== system AXI_QPSK_Tx/AXI_QPSK_Generator/M_AXIS_TIME ==
  tdata_in : Inport
  tvalid_in : Inport  Port=2
  tlast_in : Inport  Port=3
  tready_in : Inport  Port=4
  m_time_axis_tdata : xbsIndex_r4/Gateway Out  inherit_from_input=on  hdl_port=on  rows=1  columns=1  UseAsDAC=off  DACChannel='1'  interface=None  automatic_assignment=on  address_offset=hex2dec('00')  intf_name=''  intf_description=''  timing_constraint=None  locs_specified=off  LOCs={}  io_standard={}  block_type=gatewayout
  m_time_axis_tlast : xbsIndex_r4/Gateway Out  inherit_from_input=off  hdl_port=on  rows=1  columns=1  UseAsDAC=off  DACChannel='1'  interface=None  automatic_assignment=on  address_offset=hex2dec('00')  intf_name=''  intf_description=''  timing_constraint=None  locs_specified=off  LOCs={}  io_standard={}  block_type=gatewayout
  m_time_axis_tready : xbsIndex_r4/Gateway In  gui_display_data_type=Boolean  arith_type=Boolean  n_bits=16  bin_pt=14  preci_type=Single  exp_width=8  frac_width=24  rows=1  columns=1  quantization="Round  (unbiased: +/- Inf)"  overflow=Saturate  period=1/(fCIC)  UseAsADC=off  ADCChannel='1'  interface=None  automatic_assignment=on  address_offset=hex2dec('00')  intf_name=''  intf_description=''  default_value=0  timing_constraint=None  locs_specified=off  LOCs={}  io_standard={}  inherit_from_input=off  hdl_port=on  dbl_ovrd=off  block_type=gatewayin
  m_time_axis_tvalid : xbsIndex_r4/Gateway Out  inherit_from_input=off  hdl_port=on  rows=1  columns=1  UseAsDAC=off  DACChannel='1'  interface=None  automatic_assignment=on  address_offset=hex2dec('00')  intf_name=''  intf_description=''  timing_constraint=None  locs_specified=off  LOCs={}  io_standard={}  block_type=gatewayout
  tdata_out : Outport  VectorParamsAs1DForOutWhenUnconnected=off
  tvalid_out : Outport  Port=2  VectorParamsAs1DForOutWhenUnconnected=off
  tlast_out : Outport  Port=3  VectorParamsAs1DForOutWhenUnconnected=off
  tready_out : Outport  Port=4  VectorParamsAs1DForOutWhenUnconnected=off
  wires:
  tready_in/1 -> m_time_axis_tready/1
  m_time_axis_tdata/1 -> tdata_out/1
  tdata_in/1 -> m_time_axis_tdata/1
  m_time_axis_tvalid/1 -> tvalid_out/1
  tvalid_in/1 -> m_time_axis_tvalid/1
  m_time_axis_tready/1 -> tready_out/1
  m_time_axis_tlast/1 -> tlast_out/1
  tlast_in/1 -> m_time_axis_tlast/1

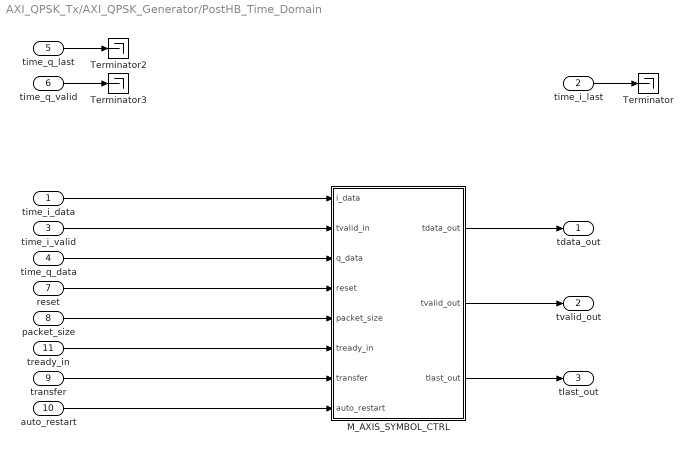
== system AXI_QPSK_Tx/AXI_QPSK_Generator/PostHB_Time_Domain ==
  time_i_data : Inport
  time_i_last : Inport  Port=2
  time_i_valid : Inport  Port=3
  time_q_data : Inport  Port=4
  time_q_last : Inport  Port=5
  time_q_valid : Inport  Port=6
  reset : Inport  Port=7
  packet_size : Inport  Port=8
  transfer : Inport  Port=9
  auto_restart : Inport  Port=10
  tready_in : Inport  Port=11
  M_AXIS_SYMBOL_CTRL : Subsystem
  Terminator : Terminator
  Terminator2 : Terminator
  Terminator3 : Terminator
  tdata_out : Outport  VectorParamsAs1DForOutWhenUnconnected=off
  tvalid_out : Outport  Port=2  VectorParamsAs1DForOutWhenUnconnected=off
  tlast_out : Outport  Port=3  VectorParamsAs1DForOutWhenUnconnected=off
  wires:
  auto_restart/1 -> M_AXIS_SYMBOL_CTRL/8(auto_restart)
  transfer/1 -> M_AXIS_SYMBOL_CTRL/7(transfer)
  M_AXIS_SYMBOL_CTRL/3(tlast_out) -> tlast_out/1
  M_AXIS_SYMBOL_CTRL/2(tvalid_out) -> tvalid_out/1
  M_AXIS_SYMBOL_CTRL/1(tdata_out) -> tdata_out/1
  tready_in/1 -> M_AXIS_SYMBOL_CTRL/6(tready_in)
  packet_size/1 -> M_AXIS_SYMBOL_CTRL/5(packet_size)
  reset/1 -> M_AXIS_SYMBOL_CTRL/4(reset)
  time_q_data/1 -> M_AXIS_SYMBOL_CTRL/3(q_data)
  time_i_valid/1 -> M_AXIS_SYMBOL_CTRL/2(tvalid_in)
  time_i_data/1 -> M_AXIS_SYMBOL_CTRL/1(i_data)
  time_q_valid/1 -> Terminator3/1
  time_q_last/1 -> Terminator2/1
  time_i_last/1 -> Terminator/1

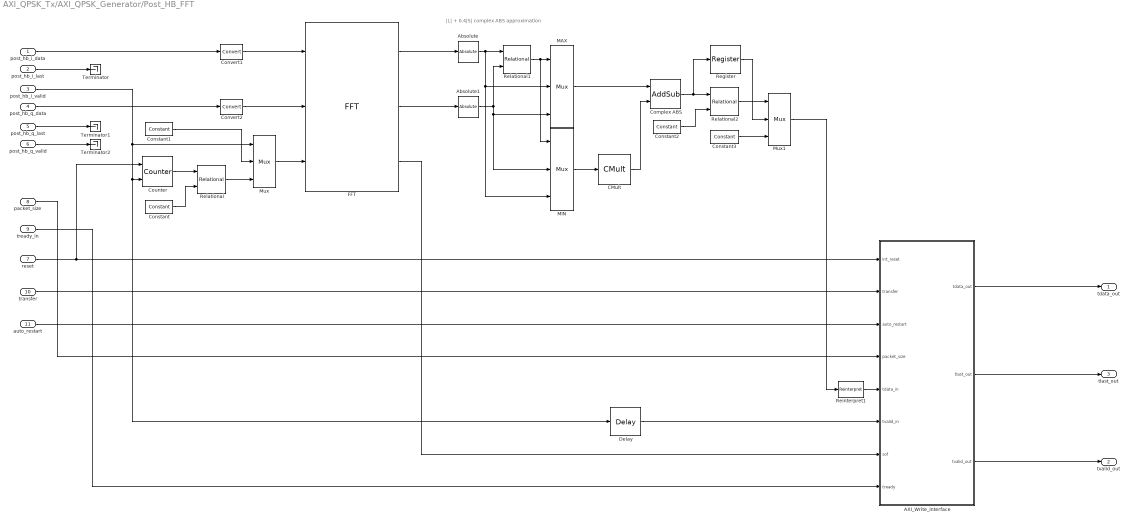
== system AXI_QPSK_Tx/AXI_QPSK_Generator/Post_HB_FFT ==
  note: |L| + 0.4|S| complex ABS approximation
  post_hb_i_data : Inport
  post_hb_i_last : Inport  Port=2
  post_hb_i_valid : Inport  Port=3
  post_hb_q_data : Inport  Port=4
  post_hb_q_last : Inport  Port=5
  post_hb_q_valid : Inport  Port=6
  reset : Inport  Port=7
  packet_size : Inport  Port=8
  tready_in : Inport  Port=9
  transfer : Inport  Port=10
  auto_restart : Inport  Port=11
  AXI_Write_Interface : Subsystem
  Absolute : xbsIndex_r4/Absolute  precision=User Defined  arith_type=Unsigned  n_bits=32  bin_pt=31  quantization=Truncate  overflow=Wrap  en=off  latency=1  dbl_ovrd=off  block_type=abs
  Absolute1 : xbsIndex_r4/Absolute  precision=User Defined  arith_type=Unsigned  n_bits=32  bin_pt=31  quantization=Truncate  overflow=Wrap  en=off  latency=1  dbl_ovrd=off  block_type=abs
  CMult : xbsIndex_r4/CMult  const=0.4  gui_display_data_type=Fixed-point  const_n_bits=32  const_bin_pt=31  float_type=Single  exp_bits=8  fraction_bits=24  en=off  latency=0  precision=Full  arith_type=Unsigned  n_bits=15  bin_pt=15  quantization=Truncate  overflow=Wrap  use_behavioral_HDL=off  mem_type=Distributed RAM  pipeline=off  dbl_ovrd=off  block_type=cmult
  Complex ABS : xbsIndex_r4/AddSub  mode=Addition  use_carryin=off  use_carryout=off  en=off  latency=1  precision=User Defined  arith_type=Unsigned  n_bits=32  bin_pt=31  quantization=Truncate  overflow=Wrap  use_behavioral_HDL=off  hw_selection=Fabric  pipelined=off  dbl_ovrd=off  block_type=addsub
  Constant : xbsIndex_r4/Constant  const=0  gui_display_data_type=Fixed-point  arith_type=Unsigned  n_bits=10  bin_pt=0  preci_type=Single  exp_width=8  frac_width=24  explicit_period=on  period=1/fHB  equ=P=C  opselect=C  inp2=PCIN>>17  opr=+  inp1=P  carry=CIN  dbl_ovrd=off  block_type=constant
  Constant1 : xbsIndex_r4/Constant  const=0  gui_display_data_type=Boolean  arith_type=Boolean  n_bits=10  bin_pt=0  preci_type=Single  exp_width=8  frac_width=24  explicit_period=on  period=1/fHB  equ=P=C  opselect=C  inp2=PCIN>>17  opr=+  inp1=P  carry=CIN  dbl_ovrd=off  block_type=constant
  Constant2 : xbsIndex_r4/Constant  const=0  gui_display_data_type=Fixed-point  arith_type=Unsigned  n_bits=32  bin_pt=31  preci_type=Single  exp_width=8  frac_width=24  explicit_period=on  period=1/fHB  equ=P=C  opselect=C  inp2=PCIN>>17  opr=+  inp1=P  carry=CIN  dbl_ovrd=off  block_type=constant
  Constant3 : xbsIndex_r4/Constant  const=2^-31  gui_display_data_type=Fixed-point  arith_type=Unsigned  n_bits=32  bin_pt=31  preci_type=Single  exp_width=8  frac_width=24  explicit_period=on  period=1/fHB  equ=P=C  opselect=C  inp2=PCIN>>17  opr=+  inp1=P  carry=CIN  dbl_ovrd=off  block_type=constant
  Convert1 : xbsIndex_r4/Convert  gui_display_data_type=Fixed-point  arith_type="Signed  (2's comp)"  n_bits=32  bin_pt=31  float_type=Single  exp_bits=8  fraction_bits=24  quantization=Truncate  overflow=Wrap  en=off  latency=0  pipeline=off  dbl_ovrd=off  block_type=convert
  Convert2 : xbsIndex_r4/Convert  gui_display_data_type=Fixed-point  arith_type="Signed  (2's comp)"  n_bits=32  bin_pt=31  float_type=Single  exp_bits=8  fraction_bits=24  quantization=Truncate  overflow=Wrap  en=off  latency=0  pipeline=off  dbl_ovrd=off  block_type=convert
  Counter : xbsIndex_r4/Counter  cnt_type=Count Limited  cnt_to=1023  operation=Up  start_count=0  cnt_by_val=1  arith_type=Unsigned  n_bits=10  bin_pt=0  load_pin=off  rst=on  en=on  explicit_period=on  period=1/fHB  use_behavioral_HDL=off  implementation=Fabric  dbl_ovrd=off  block_type=counter
  Delay : xbsIndex_r4/Delay  rst=off  infoeditControl=Selection of Reset will increase slice count due to use of real FFs and instead of SRLs  en=off  latency=2180+4  reg_retiming=off  dbl_ovrd=off  block_type=delay
  FFT : xbsIndex_r4/FFT  infoeditControl=Hardware notes: This block implements a burst IO radix-2 architecture if the <b><i>Optimize for</i></b> parameter is selected as <b><i>Resources</i></b>, and the input sample period is 8 times slower than the system sample period; otherwise a pipeline streaming architecture will be used.  transform_length=1024  scale_result_by_fft_length=on  bit_reversed_order=on  optimizegoal=Performance  start_frame=on  simulation_type=fast_sim  simulation_model=sysgen:ForwardFFT_Macro  latency=1  block_type=xfft_forward
  MAX : xbsIndex_r4/Mux  inputs=2  en=off  latency=1  precision=Full  arith_type=Unsigned  n_bits=16  bin_pt=14  quantization=Truncate  overflow=Wrap  dbl_ovrd=off  block_type=mux
  MIN : xbsIndex_r4/Mux  inputs=2  en=off  latency=1  precision=Full  arith_type=Unsigned  n_bits=16  bin_pt=14  quantization=Truncate  overflow=Wrap  dbl_ovrd=off  block_type=mux
  Mux : xbsIndex_r4/Mux  inputs=2  en=off  latency=0  precision=Full  arith_type=Unsigned  n_bits=16  bin_pt=14  quantization=Truncate  overflow=Wrap  dbl_ovrd=off  block_type=mux
  Mux1 : xbsIndex_r4/Mux  inputs=2  en=off  latency=0  precision=Full  arith_type=Unsigned  n_bits=16  bin_pt=14  quantization=Truncate  overflow=Wrap  dbl_ovrd=off  block_type=mux
  Register : xbsIndex_r4/Register  init=0  rst=off  en=off  dbl_ovrd=off  block_type=register
  Reinterpret1 : xbsIndex_r4/Reinterpret  force_arith_type=on  arith_type=Unsigned  force_bin_pt=on  bin_pt=0  block_type=reinterpret
  Relational : xbsIndex_r4/Relational  mode=a=b  op_type=Bool  en=off  latency=0  dbl_ovrd=off  block_type=relational
  Relational1 : xbsIndex_r4/Relational  mode=a<b  op_type=Bool  en=off  latency=0  dbl_ovrd=off  block_type=relational
  Relational2 : xbsIndex_r4/Relational  mode=a=b  op_type=Bool  en=off  latency=1  dbl_ovrd=off  block_type=relational
  Terminator : Terminator
  Terminator1 : Terminator
  Terminator2 : Terminator
  tdata_out : Outport  VectorParamsAs1DForOutWhenUnconnected=off
  tvalid_out : Outport  Port=2  VectorParamsAs1DForOutWhenUnconnected=off
  tlast_out : Outport  Port=3  VectorParamsAs1DForOutWhenUnconnected=off
  wires:
  post_hb_i_last/1 -> Terminator/1
  post_hb_q_last/1 -> Terminator1/1
  post_hb_q_valid/1 -> Terminator2/1
  AXI_Write_Interface/3(tvalid_out) -> tvalid_out/1
  AXI_Write_Interface/2(tlast_out) -> tlast_out/1
  packet_size/1 -> AXI_Write_Interface/4(packet_size)
  post_hb_i_valid/1 -> Delay/1, Counter/2, Mux/1
  Delay/1 -> AXI_Write_Interface/6(tvalid_in)
  reset/1 -> Counter/1, AXI_Write_Interface/1(int_reset)
  Counter/1 -> Relational/1
  Constant/1 -> Relational/2
  Mux/1 -> FFT/3
  Relational/1 -> Mux/3
  Constant1/1 -> Mux/2
  FFT/1 -> Absolute/1
  Relational1/1 -> MAX/1, MIN/1
  CMult/1 -> Complex ABS/2
  MAX/1 -> Complex ABS/1
  MIN/1 -> CMult/1
  Absolute1/1 -> MIN/2, MAX/3, Relational1/2
  Absolute/1 -> MAX/2, MIN/3, Relational1/1
  FFT/2 -> Absolute1/1
  post_hb_i_data/1 -> Convert1/1
  AXI_Write_Interface/1(tdata_out) -> tdata_out/1
  transfer/1 -> AXI_Write_Interface/2(transfer)
  auto_restart/1 -> AXI_Write_Interface/3(auto_restart)
  FFT/3 -> AXI_Write_Interface/7(sof)
  tready_in/1 -> AXI_Write_Interface/8(tready)
  post_hb_q_data/1 -> Convert2/1
  Convert1/1 -> FFT/1
  Convert2/1 -> FFT/2
  Complex ABS/1 -> Register/1, Relational2/1
  Constant2/1 -> Relational2/2
  Relational2/1 -> Mux1/1
  Constant3/1 -> Mux1/3
  Register/1 -> Mux1/2
  Mux1/1 -> Reinterpret1/1
  Reinterpret1/1 -> AXI_Write_Interface/5(tdata_in)

== system AXI_QPSK_Tx/AXI_QPSK_Generator/QPSK_symbol_mapper ==
  note: Symbol rate =
      | 500sps
  Bit_pairs : Inport
  tlast_in : Inport  Port=2
  Reset : Inport  Port=3
  tready : Inport  Port=4
  Constant : xbsIndex_r4/Constant  const=1.0  gui_display_data_type=Fixed-point  arith_type=Signed (2's comp)  n_bits=2  bin_pt=0  preci_type=Single  exp_width=8  frac_width=24  explicit_period=on  period=2/Rb  equ=P=C  opselect=C  inp2=PCIN>>17  opr=+  inp1=P  carry=CIN  dbl_ovrd=off  block_type=constant
  Constant1 : xbsIndex_r4/Constant  const=-1  gui_display_data_type=Fixed-point  arith_type=Signed (2's comp)  n_bits=2  bin_pt=0  preci_type=Single  exp_width=8  frac_width=24  explicit_period=on  period=2/Rb  equ=P=C  opselect=C  inp2=PCIN>>17  opr=+  inp1=P  carry=CIN  dbl_ovrd=off  block_type=constant
  Constant2 : xbsIndex_r4/Constant  const=1.0  gui_display_data_type=Fixed-point  arith_type=Signed (2's comp)  n_bits=2  bin_pt=0  preci_type=Single  exp_width=8  frac_width=24  explicit_period=on  period=2/Rb  equ=P=C  opselect=C  inp2=PCIN>>17  opr=+  inp1=P  carry=CIN  dbl_ovrd=off  block_type=constant
  Constant3 : xbsIndex_r4/Constant  const=-1  gui_display_data_type=Fixed-point  arith_type=Signed (2's comp)  n_bits=2  bin_pt=0  preci_type=Single  exp_width=8  frac_width=24  explicit_period=on  period=2/Rb  equ=P=C  opselect=C  inp2=PCIN>>17  opr=+  inp1=P  carry=CIN  dbl_ovrd=off  block_type=constant
  Mux : xbsIndex_r4/Mux  inputs=4  en=off  latency=0  precision=User Defined  arith_type="Signed  (2's comp)"  n_bits=2  bin_pt=0  quantization=Truncate  overflow=Wrap  dbl_ovrd=off  block_type=mux
  Mux1 : xbsIndex_r4/Mux  inputs=4  en=off  latency=0  precision=User Defined  arith_type="Signed  (2's comp)"  n_bits=2  bin_pt=0  quantization=Truncate  overflow=Wrap  dbl_ovrd=off  block_type=mux
  Register : xbsIndex_r4/Register  init=0  rst=on  en=on  dbl_ovrd=off  block_type=register
  Register1 : xbsIndex_r4/Register  init=0  rst=on  en=on  dbl_ovrd=off  block_type=register
  Register2 : xbsIndex_r4/Register  init=0  rst=on  en=on  dbl_ovrd=off  block_type=register
  I_symbols : Outport  VectorParamsAs1DForOutWhenUnconnected=off
  Q_symbols : Outport  Port=2  VectorParamsAs1DForOutWhenUnconnected=off
  tlast_out : Outport  Port=3  VectorParamsAs1DForOutWhenUnconnected=off
  wires:
  Constant/1 -> Mux/3, Mux/2
  Constant3/1 -> Mux1/3, Mux1/5
  Register/1 -> I_symbols/1
  Bit_pairs/1 -> Mux/1, Mux1/1
  Constant2/1 -> Mux1/4, Mux1/2
  Mux/1 -> Register/1
  Mux1/1 -> Register1/1
  Constant1/1 -> Mux/5, Mux/4
  Register1/1 -> Q_symbols/1
  Reset/1 -> Register2/2, Register/2, Register1/2
  tready/1 -> Register/3, Register1/3, Register2/3
  tlast_in/1 -> Register2/1
  Register2/1 -> tlast_out/1

== system AXI_QPSK_Tx/AXI_QPSK_Generator/RF_Output ==
  rf_i_data : Inport
  rf_i_valid : Inport  Port=2
  rf_i_last : Inport  Port=3
  rf_q_data : Inport  Port=4
  rf_q_valid : Inport  Port=5
  rf_q_last : Inport  Port=6
  Concat : xbsIndex_r4/Concat  num_inputs=2  dbl_ovrd=off  block_type=concat
  Logical1 : xbsIndex_r4/Logical  logical_function=AND  inputs=2  en=off  latency=0  precision=Full  arith_type=Unsigned  n_bits=16  bin_pt=0  align_bp=on  dbl_ovrd=off  block_type=logical
  Logical2 : xbsIndex_r4/Logical  logical_function=AND  inputs=2  en=off  latency=0  precision=Full  arith_type=Unsigned  n_bits=16  bin_pt=0  align_bp=on  dbl_ovrd=off  block_type=logical
  Out1 : Outport  VectorParamsAs1DForOutWhenUnconnected=off
  Out2 : Outport  Port=2  VectorParamsAs1DForOutWhenUnconnected=off
  Out3 : Outport  Port=3  VectorParamsAs1DForOutWhenUnconnected=off
  wires:
  rf_q_data/1 -> Concat/1
  Concat/1 -> Out1/1
  rf_i_last/1 -> Logical2/1
  rf_q_valid/1 -> Logical1/2
  rf_i_valid/1 -> Logical1/1
  Logical2/1 -> Out3/1
  rf_q_last/1 -> Logical2/2
  Logical1/1 -> Out2/1
  rf_i_data/1 -> Concat/2
